simulink subsystem "Piero_Hardware"  (R2023b)
settings: Solver=VariableStepAuto  StartTime=0.0  StopTime=10.0  RelTol=1e-3
settings Model: Creator=marqu  LastModifiedBy=marqu

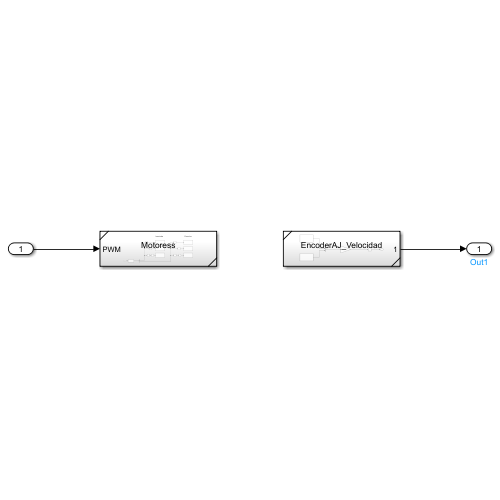
[thumbnail: Simulink's stored preview of the top-level diagram]
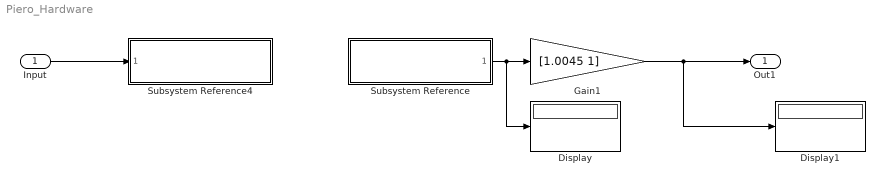
== system Piero_Hardware ==
  Input : Inport  OutDataTypeStr=int16
  Display : Display
  Display1 : Display
  Gain1 : Gain  Gain=[1.0045 1]
  Subsystem Reference : Subsystem  ReferencedSubsystem=EncoderAJ_Velocidad
  Subsystem Reference4 : Subsystem  ReferencedSubsystem=Motoress
  Out1 : Outport
  wires:
  Input/1 -> Subsystem Reference4/1
  Subsystem Reference/1 -> Gain1/1, Display/1
  Gain1/1 -> Out1/1, Display1/1
